simulink model "ballbeam_sim"  (R2014a)
settings: Solver=ode45  StartTime=0.0  StopTime=10  RelTol=1e-3
InitFcn:
  | param
undefined symbols (not defined in the file or in its folder): AP, ballbeam_ctrlss, drawBallBeam, P
settings Model: Creator=beard  LastModifiedBy=jhl48
settings DataIOCC: SignalLoggingSaveFormat=ModelDataLogs
settings OptimizationCC: ExpressionDepthLimit=2147483647  InitFltsAndDblsToZero=on
settings DebuggingCC: UnderspecifiedInitializationDetection=Classic  MultiTaskDSMMsg=warning  MultiTaskCondExecSysMsg=none  FcnCallInpInsideContextMsg=UseLocalSettings  StateNameClashWarn=warning
settings RTWCC: IncludeERTFirstTime=on
settings GRTTargetCC: CombineOutputUpdateFcns=off  GRTInterface=on

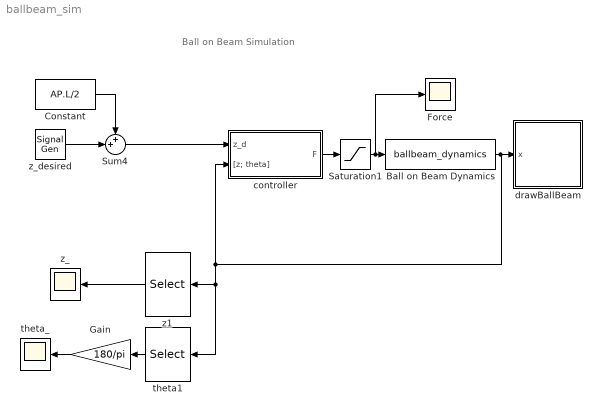
== system ballbeam_sim ==
  note: Ball on Beam Simulation
  Ball on Beam Dynamics : S-Function  FunctionName=ballbeam_dynamics  Parameters=AP  EnableBusSupport=off
  Constant : Constant  Value=AP.L/2
  Force : Scope
      settings: TimeRange=100  YMin=5  YMax=18
  Gain : Gain  Gain=180/pi
  Saturation1 : Saturate  UpperLimit=AP.F_max  LowerLimit=-AP.F_max
  Sum4 : Sum  Inputs=++|
  controller : Subsystem
  drawBallBeam : Subsystem
      mask init:
      | % drawing parameters
      | L = 0.5;
      | R = .03;
      mask Display: image(imread('tv.jpg'))
  theta1 : Selector  InputPortWidth=4  Indices=[2]
  theta_ : Scope
      settings: TimeRange=100  YMin=-3  YMax=6.5
  z1 : Selector  InputPortWidth=4  Indices=[1]
  z_ : Scope
      settings: TimeRange=100  YMin=0.025  YMax=0.475  SaveName=ScopeData2
  z_desired : SignalGenerator  WaveForm=square  Amplitude=0.125  Frequency=.02
  wires:
  Ball on Beam Dynamics/1 -> z1/1, theta1/1, controller/2("[z; theta]"), drawBallBeam/1(x)
  z_desired/1 -> Sum4/2
  Constant/1 -> Sum4/1
  Sum4/1 -> controller/1(z_d)
  z1/1 -> z_/1
  Gain/1 -> theta_/1
  theta1/1 -> Gain/1
  controller/1(F) -> Saturation1/1
  Saturation1/1 -> Force/1, Ball on Beam Dynamics/1

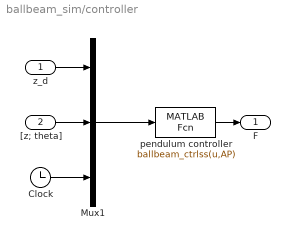
== system ballbeam_sim/controller ==
  z_d : Inport
  "[z; theta]" : Inport  Port=2
  Clock : Clock
  Mux1 : Mux  Inputs=3
  pendulum controller : MATLABFcn  MATLABFcn=ballbeam_ctrlss(u,AP)  OutputDimensions=1  SampleTime=P.Ts
  F : Outport
  wires:
  Clock/1 -> Mux1/3
  pendulum controller/1 -> F/1
  "[z; theta]"/1 -> Mux1/2
  z_d/1 -> Mux1/1
  Mux1/1 -> pendulum controller/1

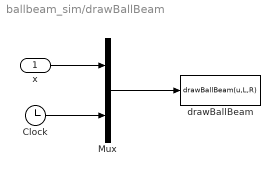
== system ballbeam_sim/drawBallBeam ==
  x : Inport
  Clock : Clock
  Mux : Mux  Inputs=2
  drawBallBeam : MATLABFcn  MATLABFcn=drawBallBeam(u,L,R)  OutputDimensions=0  SampleTime=0.1
  wires:
  Mux/1 -> drawBallBeam/1
  x/1 -> Mux/1
  Clock/1 -> Mux/2
